simulink model "SimulinkCharge_2Connect"  (R2022b)
settings: Solver=VariableStepAuto  StartTime=0.0  StopTime=300000  RelTol=1e-3
undefined symbols (not defined in the file): Ion, Lithium
libraries: spsIdealSwitchLib x4, spsBatteryLib x1, spsCurrentMeasurementLib x1, spsDCVoltageSourceLib x1, spsSeriesRLCBranchLib x1, spsVoltageMeasurementLib x1, spspowerguiLib x1
settings Model: Creator=sanan  LastModifiedBy=minar

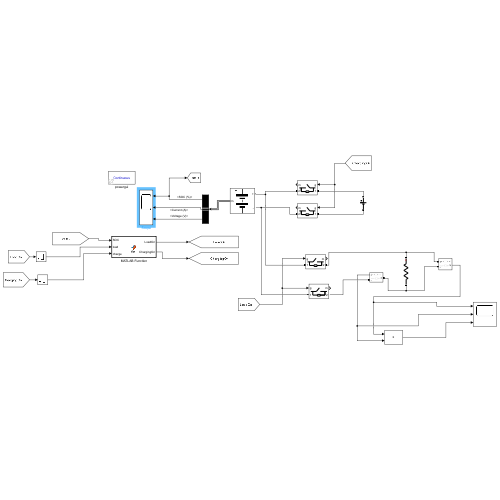
[thumbnail: Simulink's stored preview of the top-level diagram]
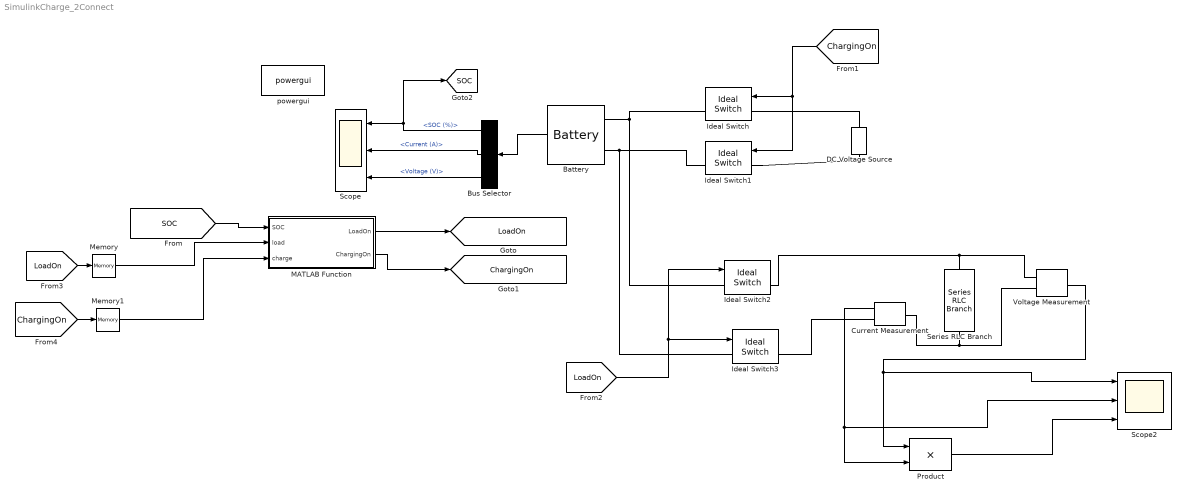
== system SimulinkCharge_2Connect ==
  Battery : spsBatteryLib/Battery  BatType=Lithium-Ion  ShowTempParam=off  ThermalPreset=no  ShowAgeParam=off  NomV=3.6  NomQ=25  SOC=80  Batt_Tr=30  PresetModel=on  MaxQ=25  MinV=2.7  FullV=4.1904  Dis_rate=10.8696  R=0.00144  Normal_OP=22.6087  expZone="[3.8894      1.2283]"  current=[6.5 13 32.5]  Units=Time  Tci=20  NomT=20  T2=-30  MaxQ2=4.8  FullV2=7.1  Normal_OP2=5.655  expZone2="[6.58           1]"  Rca=0.6  ti=2000  Dp=0  Neq0=0  Tsim=1e6  Ta1=25  Qeol=5.4*0.9  Reol=0.013333*1.2  Char_age=[2.3478, 3]  Dis_age=[2.3478, 10]  N1=1500  N2=10500  N3=1000  N4=1400  Ta2=45  N5=950
  Bus Selector : BusSelector  OutputSignals=SOC (%),Current (A),Voltage (V)
  Current Measurement : spsCurrentMeasurementLib/Current Measurement  PhasorSimulation=off  OutputType=Complex  PSBequivalent=0
  DC Voltage Source : spsDCVoltageSourceLib/DC Voltage Source  Amplitude=4  Measurements=None
  Ideal Switch{,1..3} (4 alike) : spsIdealSwitchLib/Ideal Switch  Ron=0.001  Lon=0  IC=0  Rs=1e5  Cs=inf  Measurements=on
  MATLAB Function : MATLAB Function  TreatAsAtomicUnit=on
  Memory : Memory
  Memory1 : Memory
  Product : Product
  Scope : Scope  NumInputPorts=3
  Scope2 : Scope  NumInputPorts=3
  Series RLC Branch : spsSeriesRLCBranchLib/Series RLC Branch  LConnTagsString=__new0  RConnTagsString=__new0  BranchType=R  Resistance=10  Inductance=1e-3  SetiL0=off  InitialCurrent=0  Capacitance=1e-6  Setx0=off  InitialVoltage=0  Measurements=None
  Voltage Measurement : spsVoltageMeasurementLib/Voltage Measurement  PhasorSimulation=off  OutputType=Complex  PSBequivalent=0
  powergui : spspowerguiLib/powergui  Priority=1  SimulationMode=Continuous  SampleTime=50e-6  frequency=60  Iterations=50  frequencyindice=0  Pbase=100e6  ErrMax=1e-4  UnitsV=kV  UnitsW=MW  buscounter=0  FunctionMessages=off  echomessages=off  EnableUseOfTLC=off  CurrentSourceSwitches=off  DisableSnubberDevices=off  DisableRonSwitches=off  DisableVfSwitches=off  DisplayEquations=off  AutomaticDiscreteSolvers=off  SolverType=Tustin/Backward Euler (TBE)  Interpol=off  ExternalGateDelay=off  methode=off  Ts=100  x0status=blocks  SPID=on  SwTol=0  HookPort=off  NonlinearTolerance=1e-4  nMaxIteration=100  ContinueOnMaxIteration=off  RestoreLinks=warning  ResistiveCurrentMeasurement=off  Frange=[0:2:500]  Ylog=off  Xlog=on  ShowGrid=off  save=off  variable=ZData  structure=0  ZoomFFT=off  StartTime=0.0  cycles=1  DisplayStyle=1  fundamental=60  FreqAxis=off  MaxFrequency=1000  frequencyindicesteady=1  RmsSteady=1  display=off
  tag scope: ChargingOn=global, LoadOn=global, SOC=global
  wires:
  Current Measurement/1 -> Scope2/2, Product/2
  Product/1 -> Scope2/3
  Bus Selector/2 -> Scope/2  "<Current (A)>"
  [SOC] -> MATLAB Function/1(SOC)
  [LoadOn] -> Ideal Switch3/1, Ideal Switch2/1
  Bus Selector/3 -> Scope/3  "<Voltage (V)>"
  Voltage Measurement/1 -> Scope2/1, Product/1
  [ChargingOn] -> Ideal Switch1/1, Ideal Switch/1
  Bus Selector/1 -> [SOC], Scope/1  "<SOC (%)>"
  Battery/1 -> Bus Selector/1
  [LoadOn] -> Memory/1
  [ChargingOn] -> Memory1/1
  MATLAB Function/1(LoadOn) -> [LoadOn]
  MATLAB Function/2(ChargingOn) -> [ChargingOn]
  Memory/1 -> MATLAB Function/2(load)
  Memory1/1 -> MATLAB Function/3(charge)
  connections:
  Series RLC Branch/LConn1 -- Ideal Switch2/RConn1 -- Voltage Measurement/LConn1
  Battery/LConn2 -- Ideal Switch3/LConn1 -- Ideal Switch1/RConn1
  Battery/LConn1 -- Ideal Switch2/LConn1 -- Ideal Switch/RConn1
  Current Measurement/LConn1 -- Series RLC Branch/RConn1 -- Voltage Measurement/LConn2
  Ideal Switch3/RConn1 -- Current Measurement/RConn1
  Ideal Switch1/LConn1 -- DC Voltage Source/LConn1
  DC Voltage Source/RConn1 -- Ideal Switch/LConn1

== matlab function SimulinkCharge_2Connect/MATLAB Function ==
  data: SOC input; LoadOn output; ChargingOn output; load input; charge input
function [LoadOn, ChargingOn] = fcn (SOC, load, charge)
    
    if (SOC >= 80)    
        LoadOn = 1;
        ChargingOn=0;
       
    elseif (SOC < 30)
        LoadOn = 0;
        ChargingOn=1;
    else
        LoadOn = load;
        ChargingOn = charge;
   
   end
end
